simulink library "hdlsllib_helper"  (R2019a)
settings: Solver=FixedStepDiscrete  StartTime=0.0  StopTime=10.0  RelTol=1e-3
values from neighbouring files (symbols this model uses):
  InputWordLength = ceil(raw_log2_InputWordLength) + 1    [hdlblkmask_cos.m]    (also in hdlblkmask_sin.m)
  XData = linspace(0, 0.25, NumDataPoints)    [hdlblkmask_cos.m]    (also in hdlblkmask_sin.m)
  YData = sin(2*pi*XData)    [hdlblkmask_cos.m]    (also in hdlblkmask_sin.m)
libraries: $bdroot x4
settings Model: Creator=The MathWorks, Inc.  LastModifiedBy=The MathWorks, Inc.
settings DataIOCC: SaveOutput=off  SaveTime=off  ReturnWorkspaceOutputs=off
settings OptimizationCC: BlockReduction=off  ConditionallyExecuteInputs=off  DefaultParameterBehavior=Inlined
settings DebuggingCC: AlgebraicLoopMsg=error  SingleTaskRateTransMsg=error  PregeneratedLibrarySubsystemCodeDiagnostic=none  StrictBusMsg=ErrorOnBusTreatedAsVector  ArithmeticOperatorsInVariantConditions=warning
settings HardwareCC: ProdBitPerPointer=32  ProdBitPerSizeT=32  ProdBitPerPtrDiffT=32  ProdLargestAtomicFloat=None  ProdIntDivRoundTo=Undefined  ProdEndianess=Unspecified  ProdWordSize=32  ProdHWDeviceType=ASIC/FPGA->ASIC/FPGA  ProdEqTarget=off
settings SFSimCC: SimUseLocalCustomCode=off
settings RTWCC: RTWUseLocalCustomCode=off
settings CodeAppCC: StateflowObjectComments=on
settings GRTTargetCC: TargetLangStandard=C89/C90 (ANSI)
settings ConfigComp: CovMetricSettings=dsw  CovHtmlReporting=on  CovSaveCumulativeToWorkspaceVar=on  CovSaveSingleToWorkspaceVar=on  CovShowResultsExplorer=off  CovExternalEMLEnable=off

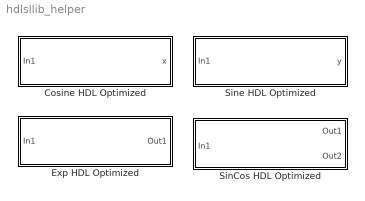
== system hdlsllib_helper ==
  Cosine HDL Optimized : Subsystem  mask{NumDataPoints=64, TableDataTypeStr=fixdt(0,16,15), SimulateLUTROMDelay=off}
      mask prompts: NumDataPoints "HDLShared:hdlshared:CosineHDL_Npts"; TableDataTypeStr "Simulink:blkprm_prompts:TABLE_UNIFIEDDATATYPE"; SimulateLUTROMDelay "HDLShared:hdlshared:CosineHDL_Map2RAM"
      mask init:
      | block_name=gcb();
      | [InputWordLength,YData,TableWordLength,TableFracLength,OutputWordLength,OutputFracLength] = hdlblkmask_cos(block_name,TableDataTypeStr,NumDataPoints);
      | 
      | gcb_lut = get_param([block_name, '/Look-Up Table'],'handle');
      | set_param(gcb_lut,'BreakpointsForDimension1FirstPoint','fi(0,0,InputWordLength,0)');
      | set_param(gcb_lut,'BreakpointsForDimension1Spacing','fi(1,0,InputWordLength,0)');
      | set_param(gcb_lut, 'IndexSearchMethod', 'Evenly spaced points');
      | 
      | SampleTime = -1;
      mask DialogControl DescGroupVar Prompt: HDLShared:hdlshared:CosineHDL_Title
      mask DialogControl DetailedDescription Prompt: HDLShared:hdlshared:CosineHDL_Description
      mask DialogControl NumDataPoints Prompt: Number of data points
      mask DialogControl TableDataTypeStr Prompt: Table data type:
      mask DialogControl SimulateLUTROMDelay Prompt: Simulate RAM Delay
      mask Display:
      | port_label('input',1,'u')
      | port_label('output',1,'cos(2*pi*u)')
      | xpos = 0.35;
      | yoffset = 0.5;
      | if ( SimulateLUTROMDelay )
      |   text(xpos,yoffset,'HDL (Z^{-1})','texmode','on')
      | else
      |    text(xpos,yoffset,'HDL')
      | end
  Exp HDL Optimized : Subsystem  mask{NumDataPoints=64, TableDataTypeStr=fixdt(0,16,15), SimulateLUTROMDelay=off}
      mask prompts: NumDataPoints "HDLShared:hdlshared:CosineHDL_Npts"; TableDataTypeStr "Simulink:blkprm_prompts:TABLE_UNIFIEDDATATYPE"; SimulateLUTROMDelay "HDLShared:hdlshared:CosineHDL_Map2RAM"
      mask TypeOptions NumDataPoints: cos_hdl/NumDataPoints | sin_hdl/NumDataPoints
      mask TypeOptions TableDataTypeStr: sin_hdl/TableDataTypeStr | cos_hdl/TableDataTypeStr
      mask TypeOptions SimulateLUTROMDelay: cos_hdl/SimulateLUTROMDelay | sin_hdl/SimulateLUTROMDelay
      mask DialogControl DescGroupVar Prompt: HDLShared:hdlshared:ExpHDL_Title
      mask DialogControl DescTextVar Prompt: HDLShared:hdlshared:ExpHDL_Description
      mask DialogControl NumDataPoints Prompt: Number of data points
      mask DialogControl TableDataTypeStr Prompt: Table data type:
      mask DialogControl SimulateLUTROMDelay Prompt: Simulate RAM Delay
      mask Display:
      | port_label('input',1,'u')
      | port_label('output',1,'exp(2*pi*u)')
      | xpos = 0.35;
      | yoffset = 0.5;
      | if ( SimulateLUTROMDelay )
      |   text(xpos,yoffset,'HDL (Z^{-1})','texmode','on')
      | else
      |    text(xpos,yoffset,'HDL')
      | end
  SinCos HDL Optimized : Subsystem  mask{NumDataPoints=64, TableDataTypeStr=fixdt(0,16,15), SimulateLUTROMDelay=off}
      mask prompts: NumDataPoints "HDLShared:hdlshared:CosineHDL_Npts"; TableDataTypeStr "Simulink:blkprm_prompts:TABLE_UNIFIEDDATATYPE"; SimulateLUTROMDelay "HDLShared:hdlshared:CosineHDL_Map2RAM"
      mask TypeOptions NumDataPoints: cos_hdl/NumDataPoints | sin_hdl/NumDataPoints
      mask TypeOptions TableDataTypeStr: sin_hdl/TableDataTypeStr | cos_hdl/TableDataTypeStr
      mask TypeOptions SimulateLUTROMDelay: cos_hdl/SimulateLUTROMDelay | sin_hdl/SimulateLUTROMDelay
      mask DialogControl DescGroupVar Prompt: HDLShared:hdlshared:ExpHDL_Title
      mask DialogControl DescTextVar Prompt: HDLShared:hdlshared:ExpHDL_Description
      mask DialogControl NumDataPoints Prompt: Number of data points
      mask DialogControl TableDataTypeStr Prompt: Table data type:
      mask DialogControl SimulateLUTROMDelay Prompt: Simulate RAM Delay
      mask Display:
      | port_label('input',1,'u')
      | port_label('output',1,'sin(2*pi*u)')
      | port_label('output',2,'cos(2*pi*u)')
      | xpos = 0.35;
      | yoffset = 0.5;
      | if ( SimulateLUTROMDelay )
      |   text(xpos,yoffset,'HDL (Z^{-1})','texmode','on')
      | else
      |    text(xpos,yoffset,'HDL')
      | end
  Sine HDL Optimized : Subsystem  mask{NumDataPoints=64, TableDataTypeStr=fixdt(0,16,15), SimulateLUTROMDelay=off}
      mask prompts: NumDataPoints "HDLShared:hdlshared:CosineHDL_Npts"; TableDataTypeStr "Simulink:blkprm_prompts:TABLE_UNIFIEDDATATYPE"; SimulateLUTROMDelay "HDLShared:hdlshared:CosineHDL_Map2RAM"
      mask init:
      | block_name=gcb();
      | [InputWordLength,YData,TableWordLength,TableFracLength,OutputWordLength,OutputFracLength] = hdlblkmask_sin(block_name,TableDataTypeStr,NumDataPoints);
      | 
      | gcb_lut = get_param([block_name, '/Look-Up Table'],'handle');
      | set_param(gcb_lut,'BreakpointsForDimension1FirstPoint','fi(0,0,InputWordLength,0)');
      | set_param(gcb_lut,'BreakpointsForDimension1Spacing','fi(1,0,InputWordLength,0)');
      | set_param(gcb_lut, 'IndexSearchMethod', 'Evenly spaced points');
      | 
      | SampleTime = -1;
      mask DialogControl DescGroupVar Prompt: HDLShared:hdlshared:SineHDL_Title
      mask DialogControl DetailedDescription Prompt: HDLShared:hdlshared:SineHDL_Description
      mask DialogControl NumDataPoints Prompt: Number of data points
      mask DialogControl TableDataTypeStr Prompt: Table data type:
      mask DialogControl SimulateLUTROMDelay Prompt: Simulate RAM Delay
      mask Display:
      | port_label('input',1,'u')
      | port_label('output',1,'sin(2*pi*u)')
      | xpos = 0.35;
      | yoffset = 0.5;
      | if ( SimulateLUTROMDelay )
      |   text(xpos,yoffset,'HDL (Z^{-1})','texmode','on')
      | else
      |    text(xpos,yoffset,'HDL')
      | end

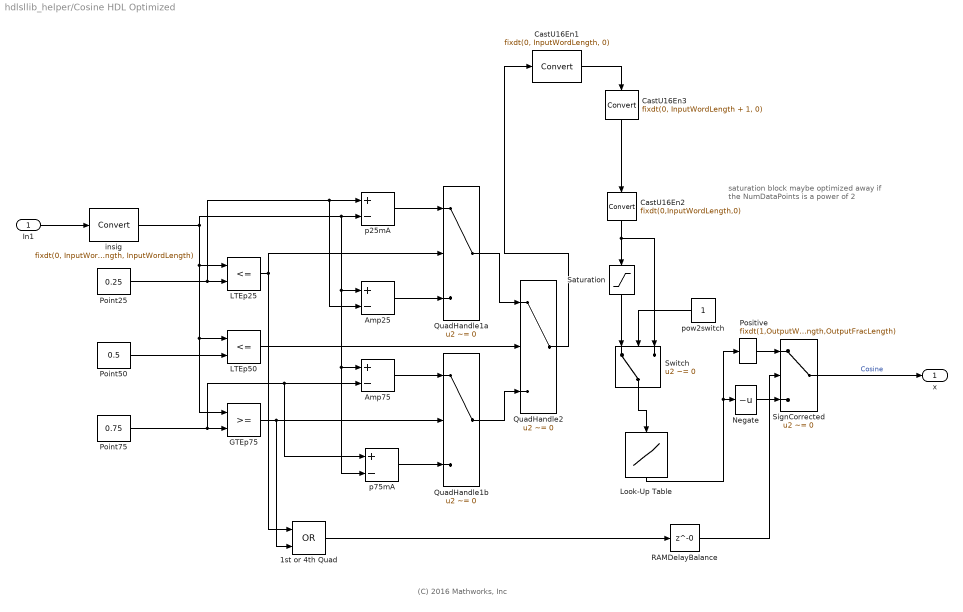
== system hdlsllib_helper/Cosine HDL Optimized ==
  note: saturation block maybe optimized away
      | if the NumDataPoints is a power of 2
  note: (C) 2016 Mathworks, Inc
  In1 : Inport
  1st or 4th Quad : Logic  Operator=OR  AllPortsSameDT=off  OutDataTypeStr=uint(8)
  Amp25 : Sum  Inputs=+-  LockScale=on
  Amp75 : Sum  Inputs=+-  LockScale=on
  CastU16En1 : DataTypeConversion  OutDataTypeStr=fixdt(0, InputWordLength, 0)  ConvertRealWorld=Stored Integer (SI)  LockScale=on
  CastU16En2 : DataTypeConversion  OutDataTypeStr=fixdt(0,InputWordLength,0)  ConvertRealWorld=Stored Integer (SI)  SaturateOnIntegerOverflow=on  LockScale=on
  CastU16En3 : DataTypeConversion  OutDataTypeStr=fixdt(0, InputWordLength + 1, 0)  LockScale=on
  GTEp75 : RelationalOperator  OutDataTypeStr=boolean  ZeroCross=off  RndMeth=Nearest
  LTEp25 : RelationalOperator  Operator=<=  OutDataTypeStr=boolean  ZeroCross=off  RndMeth=Nearest
  LTEp50 : RelationalOperator  Operator=<=  OutDataTypeStr=boolean  ZeroCross=off  RndMeth=Nearest
  Look-Up Table : Lookup_n-D  NumberOfTableDimensions=1  LookupTableObject=''  BreakpointsSpecification=Even spacing  BreakpointsForDimension1=XData  BreakpointsForDimension1FirstPoint=fi(0,0,InputWordLength,0)  BreakpointsForDimension1Spacing=fi(1,0,InputWordLength,0)  IndexSearchMethod=Evenly spaced points  Table=YData  TableDataTypeStr=fixdt(0, TableWordLength, TableFracLength)  InterpMethod=Flat  ExtrapMethod=Clip  DiagnosticForOutOfRangeInput=Error  OutDataTypeStr=fixdt(1,OutputWordLength,OutputFracLength)  InputSameDT=on  LockScale=on
  Negate : UnaryMinus
  Point25 : Constant  Value=0.25  OutDataTypeStr=fixdt(0, OutputWordLength, OutputWordLength)  SampleTime=SampleTime
  Point50 : Constant  Value=0.5  OutDataTypeStr=fixdt(0, OutputWordLength, OutputWordLength)  SampleTime=SampleTime
  Point75 : Constant  Value=0.75  OutDataTypeStr=fixdt(0, OutputWordLength, OutputWordLength)  SampleTime=SampleTime
  Positive : DataTypeConversion  OutDataTypeStr=fixdt(1,OutputWordLength,OutputFracLength)
  QuadHandle1a : Switch  Criteria=u2 ~= 0  ZeroCross=off
  QuadHandle1b : Switch  Criteria=u2 ~= 0  ZeroCross=off
  QuadHandle2 : Switch  Criteria=u2 ~= 0  OutDataTypeStr=fixdt(0,InputWordLength,InputWordLength,'DataTypeOverride','off')  ZeroCross=off  SaturateOnIntegerOverflow=on
  RAMDelayBalance : Delay  DelayLength=0
  Saturation : Saturate  UpperLimit=fi( min(NumDataPoints-1, 2^InputWordLength-1) ,0,InputWordLength,0)  LowerLimit=fi(0,0,InputWordLength,0)  LinearizeAsGain=off
  SignCorrected : Switch  Criteria=u2 ~= 0  Threshold=1  ZeroCross=off
  Switch : Switch  Criteria=u2 ~= 0
  insig : DataTypeConversion  OutDataTypeStr=fixdt(0, InputWordLength, InputWordLength)  LockScale=on
  p25mA : Sum  Inputs=+-  LockScale=on
  p75mA : Sum  Inputs=+-  LockScale=on
  pow2switch : Constant  OutDataTypeStr=boolean  SampleTime=-1
  x : Outport
  wires:
  Positive/1 -> SignCorrected/1
  pow2switch/1 -> Switch/2
  CastU16En1/1 -> CastU16En3/1
  Switch/1 -> Look-Up Table/1
  Saturation/1 -> Switch/1
  CastU16En3/1 -> CastU16En2/1
  SignCorrected/1 -> x/1  "Cosine"
  QuadHandle1a/1 -> QuadHandle2/1
  QuadHandle2/1 -> CastU16En1/1
  insig/1 -> p75mA/2, Amp75/1, Amp25/1, p25mA/2, GTEp75/1, LTEp50/1, LTEp25/1
  Point50/1 -> LTEp50/2
  In1/1 -> insig/1
  GTEp75/1 -> 1st or 4th Quad/2, QuadHandle1b/2
  1st or 4th Quad/1 -> RAMDelayBalance/1
  LTEp25/1 -> 1st or 4th Quad/1, QuadHandle1a/2
  Point25/1 -> Amp25/2, p25mA/1, LTEp25/2
  Point75/1 -> p75mA/1, Amp75/2, GTEp75/2
  Amp25/1 -> QuadHandle1a/3
  QuadHandle1b/1 -> QuadHandle2/3
  p75mA/1 -> QuadHandle1b/3
  LTEp50/1 -> QuadHandle2/2
  CastU16En2/1 -> Saturation/1, Switch/3
  Amp75/1 -> QuadHandle1b/1
  Negate/1 -> SignCorrected/3
  p25mA/1 -> QuadHandle1a/1
  Look-Up Table/1 -> Negate/1, Positive/1
  RAMDelayBalance/1 -> SignCorrected/2

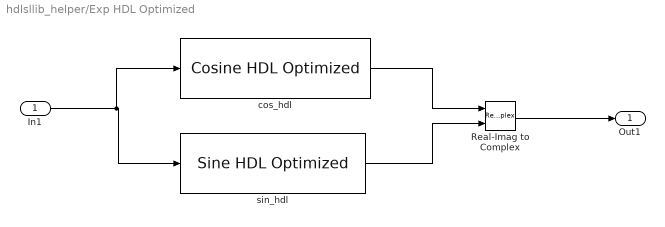
== system hdlsllib_helper/Exp HDL Optimized ==
  In1 : Inport
  Real-Imag to Complex : RealImagToComplex
  cos_hdl : $bdroot/Cosine HDL Optimized  NumDataPoints=NumDataPoints  TableDataTypeStr=fixdt(0,16,15)  SimulateLUTROMDelay=off
  sin_hdl : $bdroot/Sine HDL Optimized  NumDataPoints=NumDataPoints  TableDataTypeStr=fixdt(0,16,15)  SimulateLUTROMDelay=off
  Out1 : Outport
  wires:
  sin_hdl/1 -> Real-Imag to Complex/2
  cos_hdl/1 -> Real-Imag to Complex/1
  In1/1 -> sin_hdl/1, cos_hdl/1
  Real-Imag to Complex/1 -> Out1/1

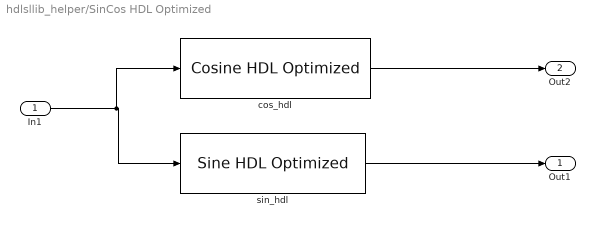
== system hdlsllib_helper/SinCos HDL Optimized ==
  In1 : Inport
  cos_hdl : $bdroot/Cosine HDL Optimized  NumDataPoints=NumDataPoints  TableDataTypeStr=fixdt(0,16,15)  SimulateLUTROMDelay=off
  sin_hdl : $bdroot/Sine HDL Optimized  NumDataPoints=NumDataPoints  TableDataTypeStr=fixdt(0,16,15)  SimulateLUTROMDelay=off
  Out1 : Outport
  Out2 : Outport  Port=2
  wires:
  sin_hdl/1 -> Out1/1
  cos_hdl/1 -> Out2/1
  In1/1 -> sin_hdl/1, cos_hdl/1

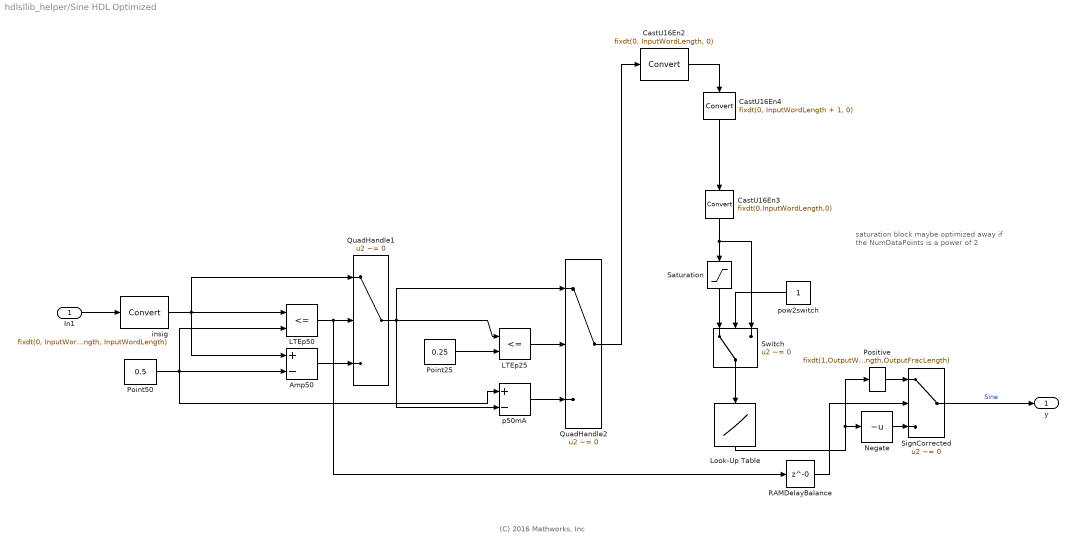
== system hdlsllib_helper/Sine HDL Optimized ==
  note: saturation block maybe optimized away
      | if the NumDataPoints is a power of 2
  note: (C) 2016 Mathworks, Inc
  In1 : Inport
  Amp50 : Sum  Inputs=+-  LockScale=on
  CastU16En2 : DataTypeConversion  OutDataTypeStr=fixdt(0, InputWordLength, 0)  ConvertRealWorld=Stored Integer (SI)  LockScale=on
  CastU16En3 : DataTypeConversion  OutDataTypeStr=fixdt(0,InputWordLength,0)  ConvertRealWorld=Stored Integer (SI)  SaturateOnIntegerOverflow=on  LockScale=on
  CastU16En4 : DataTypeConversion  OutDataTypeStr=fixdt(0, InputWordLength + 1, 0)  LockScale=on
  LTEp25 : RelationalOperator  Operator=<=  OutDataTypeStr=boolean  ZeroCross=off  RndMeth=Nearest
  LTEp50 : RelationalOperator  Operator=<=  OutDataTypeStr=boolean  ZeroCross=off  RndMeth=Nearest
  Look-Up Table : Lookup_n-D  NumberOfTableDimensions=1  LookupTableObject=''  BreakpointsSpecification=Even spacing  BreakpointsForDimension1=XData  BreakpointsForDimension1FirstPoint=fi(0,0,InputWordLength,0)  BreakpointsForDimension1Spacing=fi(1,0,InputWordLength,0)  IndexSearchMethod=Evenly spaced points  Table=YData  TableDataTypeStr=fixdt(0, TableWordLength, TableFracLength)  InterpMethod=Flat  ExtrapMethod=Clip  DiagnosticForOutOfRangeInput=Error  OutDataTypeStr=fixdt(1,OutputWordLength,OutputFracLength)  InputSameDT=on  LockScale=on
  Negate : UnaryMinus
  Point25 : Constant  Value=0.25  OutDataTypeStr=fixdt(0, OutputWordLength, OutputWordLength)  SampleTime=-1
  Point50 : Constant  Value=0.5  OutDataTypeStr=fixdt(0, OutputWordLength, OutputWordLength)  SampleTime=-1
  Positive : DataTypeConversion  OutDataTypeStr=fixdt(1,OutputWordLength,OutputFracLength)
  QuadHandle1 : Switch  Criteria=u2 ~= 0  ZeroCross=off
  QuadHandle2 : Switch  Criteria=u2 ~= 0  OutDataTypeStr=fixdt(0,InputWordLength,InputWordLength,'DataTypeOverride','off')  ZeroCross=off
  RAMDelayBalance : Delay  DelayLength=0
  Saturation : Saturate  UpperLimit=fi( min(NumDataPoints-1, 2^InputWordLength-1) ,0,InputWordLength,0)  LowerLimit=fi(0,0,InputWordLength,0)  LinearizeAsGain=off
  SignCorrected : Switch  Criteria=u2 ~= 0  Threshold=1  ZeroCross=off
  Switch : Switch  Criteria=u2 ~= 0
  insig : DataTypeConversion  OutDataTypeStr=fixdt(0, InputWordLength, InputWordLength)  LockScale=on
  p50mA : Sum  Inputs=+-  LockScale=on
  pow2switch : Constant  OutDataTypeStr=boolean  SampleTime=-1
  y : Outport
  wires:
  Positive/1 -> SignCorrected/1
  Switch/1 -> Look-Up Table/1
  pow2switch/1 -> Switch/2
  CastU16En2/1 -> CastU16En4/1
  Saturation/1 -> Switch/1
  CastU16En4/1 -> CastU16En3/1
  CastU16En3/1 -> Saturation/1, Switch/3
  SignCorrected/1 -> y/1  "Sine"
  Point50/1 -> Amp50/2, p50mA/1, LTEp50/2
  LTEp50/1 -> QuadHandle1/2, RAMDelayBalance/1
  p50mA/1 -> QuadHandle2/3
  Negate/1 -> SignCorrected/3
  insig/1 -> LTEp50/1, QuadHandle1/1, Amp50/1
  Amp50/1 -> QuadHandle1/3
  Point25/1 -> LTEp25/2
  In1/1 -> insig/1
  QuadHandle2/1 -> CastU16En2/1
  QuadHandle1/1 -> LTEp25/1, QuadHandle2/1, p50mA/2
  LTEp25/1 -> QuadHandle2/2
  Look-Up Table/1 -> Negate/1, Positive/1
  RAMDelayBalance/1 -> SignCorrected/2
